simulink model "DualBand_DualMod_Mesh_Simulink"  (R2024b)
settings: Solver=FixedStepAuto  StartTime=0.0  StopTime=210  FixedStep=1  RelTol=1e-3
settings Model: Creator=ARYA MGC  LastModifiedBy=ARYA MGC

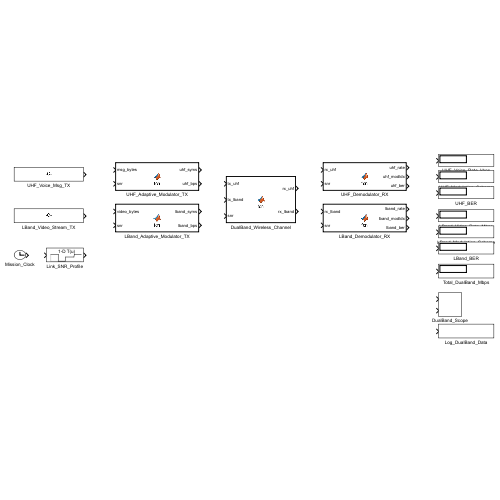
[thumbnail: Simulink's stored preview of the top-level diagram]
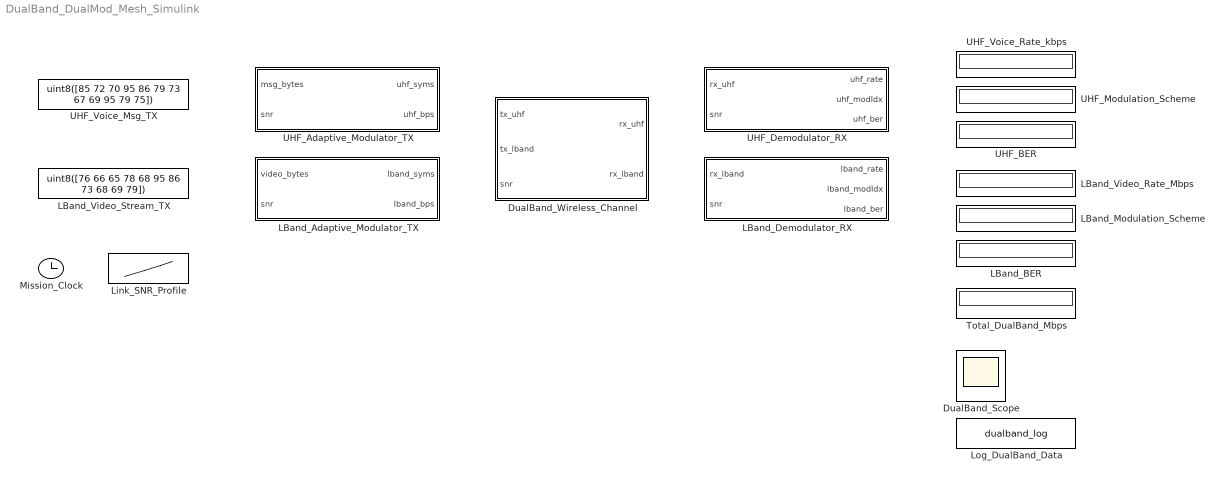
== system DualBand_DualMod_Mesh_Simulink ==
  DualBand_Scope : Scope  NumInputPorts=2
  DualBand_Wireless_Channel : MATLAB Function  TreatAsAtomicUnit=on
  LBand_Adaptive_Modulator_TX : MATLAB Function  TreatAsAtomicUnit=on
  LBand_BER : Display
  LBand_Demodulator_RX : MATLAB Function  TreatAsAtomicUnit=on
  LBand_Modulation_Scheme : Display
  LBand_Video_Rate_Mbps : Display
  LBand_Video_Stream_TX : Constant  Value=uint8([76 66 65 78 68 95 86 73 68 69 79])
  Link_SNR_Profile : Lookup_n-D  NumberOfTableDimensions=1  BreakpointsForDimension1=[0 50 51 100 101 160 161 210]  Table="[30 30 18 18  25  25  30  30]"  InternalRulePriority=Speed  RndMeth=Simplest
  Log_DualBand_Data : ToWorkspace  VariableName=dualband_log  SampleTime=-1
  Mission_Clock : Clock
  Total_DualBand_Mbps : Display
  UHF_Adaptive_Modulator_TX : MATLAB Function  TreatAsAtomicUnit=on
  UHF_BER : Display
  UHF_Demodulator_RX : MATLAB Function  TreatAsAtomicUnit=on
  UHF_Modulation_Scheme : Display
  UHF_Voice_Msg_TX : Constant  Value=uint8([85 72 70 95 86 79 73 67 69 95 79 75])
  UHF_Voice_Rate_kbps : Display

== matlab function DualBand_DualMod_Mesh_Simulink/LBand_Adaptive_Modulator_TX ==
  data: video_bytes input; lband_syms output; snr input; lband_bps output
function [lband_syms, lband_bps] = fcn(video_bytes, snr)
%% L-BAND ADAPTIVE MODULATOR (TX)
coder.extrinsic('process_lband_tx');
lband_syms = complex(zeros(1, 400)); lband_bps = 4;
[lband_syms, lband_bps] = process_lband_tx(video_bytes, snr);

== matlab function DualBand_DualMod_Mesh_Simulink/UHF_Adaptive_Modulator_TX ==
  data: msg_bytes input; uhf_syms output; snr input; uhf_bps output
function [uhf_syms, uhf_bps] = fcn(msg_bytes, snr)
%% UHF ADAPTIVE MODULATOR (TX)
coder.extrinsic('process_uhf_tx');
uhf_syms = complex(zeros(1, 400)); uhf_bps = 1;
[uhf_syms, uhf_bps] = process_uhf_tx(msg_bytes, snr);

== matlab function DualBand_DualMod_Mesh_Simulink/DualBand_Wireless_Channel ==
  data: tx_uhf input; rx_uhf output; tx_lband input; snr input; rx_lband output
function [rx_uhf, rx_lband] = fcn(tx_uhf, tx_lband, snr)
%% DUAL-BAND WIRELESS CHANNEL
coder.extrinsic('awgn');
rx_uhf = awgn(tx_uhf, snr, 'measured');
rx_lband = awgn(tx_lband, max(2, snr - 3), 'measured');

== matlab function DualBand_DualMod_Mesh_Simulink/UHF_Demodulator_RX ==
  data: rx_uhf input; uhf_rate output; snr input; uhf_modIdx output; uhf_ber output
function [uhf_rate, uhf_modIdx, uhf_ber] = fcn(rx_uhf, snr)
%% UHF DEMODULATOR (RX)
coder.extrinsic('process_uhf_rx');
uhf_rate = 0; uhf_modIdx = 1; uhf_ber = 0;
[uhf_rate, uhf_modIdx, uhf_ber] = process_uhf_rx(rx_uhf, snr);

== matlab function DualBand_DualMod_Mesh_Simulink/LBand_Demodulator_RX ==
  data: rx_lband input; lband_rate output; snr input; lband_modIdx output; lband_ber output
function [lband_rate, lband_modIdx, lband_ber] = fcn(rx_lband, snr)
%% L-BAND DEMODULATOR (RX)
coder.extrinsic('process_lband_rx');
lband_rate = 0; lband_modIdx = 3; lband_ber = 0;
[lband_rate, lband_modIdx, lband_ber] = process_lband_rx(rx_lband, snr);
